simulink model "BugE_v0_40_MAS_loads_reg"  (R2015b)
settings: Solver=FixedStepDiscrete  StartTime=0.0  StopTime=1370  FixedStep=sample_time  RelTol=1e-3
values from neighbouring files (symbols this model uses):
  AB_diode_dV = 0.9    [main_sync.m]
  air_density = 1.225    [main_sync.m]
  bus_ac_Pmax_abs = 240    [main_sync.m]
  bus_charger_Pmax = 1000    [main_sync.m]
  bus_load_Pmax_abs = 260    [main_sync.m]
  capInitVolt = capVmax*sqrt(capInitSoC)    [main_sync.m]
  cyc_kph = [cyc_kph(:,1), cyc_kph(:,2)*speed_max_limit/speed_max]    [main_sync.m]
  cyc_repeat = 0    [main_sync.m]
  ess1_init_soc = 1    [main_sync.m]
  ess1_soh = 1    [main_sync.m]
  ess2_init_soc = 1    [main_sync.m]
  ess2_soh = 1    [main_sync.m]
  ess3_init_soc = 1    [main_sync.m]
  ess3_soh = 1    [main_sync.m]
  ess4_init_soc = 1    [main_sync.m]
  ess4_soh = 1    [main_sync.m]
  ess5_init_soc = 1    [main_sync.m]
  ess5_soh = 1    [main_sync.m]
  gear_ratio = 6    [main_sync.m]
  JADE_on = 0    [main_sync.m]
  loadpower = rawcsv(:,2)    [main_sync.m]
  loadtime = rawcsv(:,1)    [main_sync.m]
  lockSOCs = 0    [main_sync.m]
  max_brk_torque = 300    [main_sync.m]
  no_wheels = 3    [main_sync.m]
  period2 = max(loadtime)    [main_sync.m]
  PV_Pmax = 100    [main_sync.m]
  sample_time = 0.01    [main_sync.m]
  startup_seq_step_delay = 0.2    [main_sync.m]
  stop_option = 0    [main_sync.m]
  use_drive_cycle = 1    [main_sync.m]
  use_real_subs_loads = 1    [main_sync.m]
  vbus_max = 25    [main_sync.m]
  vbus_min = 17    [main_sync.m]
  vbus_safety_threshold = 2    [main_sync.m]
  vbus_threshold = 20    [main_sync.m]
  veh_CD = 0.35    [main_sync.m]
  veh_FA = 1.543    [main_sync.m]
  veh_gravity = 9.81*veh_mass    (= 1863.9)    [main_sync.m]
  veh_mass = 190    [main_sync.m]
  wh_1st_rrc = 0.02    [main_sync.m]
  wh_bearing_frc = 0.0015    [main_sync.m]
  wh_inertia = 0.0556    [main_sync.m]
  wh_radius = 0.508/2    (= 0.254)    [main_sync.m]
undefined symbols (not defined in the file or in its folder): capC, capR, cyc_acc, cyc_avg_time_samples, cyc_brk, cyc_grade, cyc_key, DCM_eff_factor_for_Vin, DCM_eff_for_Iout, DCM_Iout, DCM_Iout_max, DCM_Pin_noload, DCM_Pout_max, DCM_Vin, DCM_Vout, DiscIntNeverNeededParam, ess2_coulombic_eff, ess2_Ineg_max_SOC, ess2_Ineg_max_temp, ess2_Ipos_max_SOC, ess2_Ipos_max_temp, ess2_max_ah_cap, ess2_max_volts, ess2_min_volts, ess2_module_parallel, ess2_module_series, ess2_r_dis, ess2_soc, ess2_SOC_for_Ilimit, ess2_temp_for_Ilimit, ess2_temp_max, ess2_tmp, ess2_voc, ess3_coulombic_eff, ess3_max_ah_cap, ess3_module_parallel, ess3_module_series, ess3_r_dis, ess3_soc, ess3_tmp, ess3_voc, ess_coulombic_eff, ess_Ineg_max_SOC, ess_Ineg_max_temp, ess_Ipos_max_SOC, ess_Ipos_max_temp, ess_max_ah_cap, ess_max_volts, ess_min_volts, ess_module_parallel, ess_module_series, ess_nominal_volts, ess_r_dis, ess_soc, ess_SOC_for_Ilimit, ess_temp_for_Ilimit, ess_temp_max, ess_tmp, ess_voc, MC_eff1 ... (+18)
libraries: simulink x140, commfilt2 x1, simulink_extras x1
(part 4 of 7)

== system BugE_v0_40_MAS_loads_reg/Energy Storage (New Grid)/MB2 DCDC/eff_maps ==
  "P into bus cmd " : Inport
  Vbus : Inport  Port=2
  Vbatt : Inport  Port=3
  1/V : Product  Inputs=*/
  >= eps : Saturate  UpperLimit=inf  LowerLimit=eps
  Clock : Clock
  Demux : Demux  Outputs=2
  Discrete-Time Integrator : DiscreteIntegrator  InitialConditionSetting=State (most efficient)  SampleTime=sample_time  ICPrevOutput=DiscIntNeverNeededParam  ICPrevScaledInput=DiscIntNeverNeededParam
  Discrete-Time Integrator1 : DiscreteIntegrator  InitialConditionSetting=State (most efficient)  SampleTime=sample_time  ICPrevOutput=DiscIntNeverNeededParam  ICPrevScaledInput=DiscIntNeverNeededParam
  Display : Display
  Divide : Product  Inputs=/*
  Divide1 : Product  Inputs=*/
  Gain : Gain  Gain=-1
  Interpolation: efficiency2 : Lookup_n-D  NumberOfTableDimensions=3  BreakpointsForDimension1=MC_Pouts  BreakpointsForDimension2=MC_Vins  BreakpointsForDimension3=MC_Vouts  Table=MC_eff2  InterpMethod=Cubic spline  InternalRulePriority=Speed  RndMeth=Simplest  InputSameDT=on
  Interpolation: efficiency1 : Lookup_n-D  NumberOfTableDimensions=3  BreakpointsForDimension1=MC_Pins  BreakpointsForDimension2=MC_Vins  BreakpointsForDimension3=MC_Vouts  Table=MC_eff1  InterpMethod=Cubic spline  InternalRulePriority=Speed  RndMeth=Simplest  InputSameDT=on
  Mux : Mux  Inputs=2
  Mux1 : Mux  Inputs=2
  Mux2 : Mux  Inputs=2
  P from batt : Switch
  P from batt1 : Switch
  Product : Product
  Saturation : Saturate  UpperLimit=MC_max_eff  LowerLimit=eps
  Saturation1 : Saturate  UpperLimit=MC_max_eff  LowerLimit=eps
  Saturation2 : Saturate  UpperLimit=inf  LowerLimit=eps
  Subtract : Sum  Inputs=+-
  Switch1 : Switch
  avg eff : Display
  I from batt & into bus : Outport
  wires:
  Vbatt/1 -> Mux/2, Mux1/1
  Demux/2 -> Interpolation: efficiency1/3, Interpolation: efficiency2/3
  Mux/1 -> Switch1/3
  Switch1/1 -> Demux/1
  Gain/1 -> Interpolation: efficiency1/1
  Divide/1 -> P from batt/1
  Interpolation: efficiency1/1 -> Saturation1/1
  Product/1 -> P from batt/3
  Mux2/1 -> 1/V/1
  Mux1/1 -> >= eps/1, Switch1/1
  1/V/1 -> I from batt & into bus/1
  >= eps/1 -> 1/V/2
  Demux/1 -> Interpolation: efficiency2/2, Interpolation: efficiency1/2
  Vbus/1 -> Mux1/2, Mux/1
  Saturation/1 -> Divide/1
  P from batt/1 -> Subtract/1, Mux2/1
  Subtract/1 -> Discrete-Time Integrator/1
  Discrete-Time Integrator/1 -> Display/1  "E lost MB2 DCDC"
  Interpolation: efficiency2/1 -> P from batt1/1, Saturation/1
  "P into bus cmd "/1 -> Subtract/2, Gain/1, Interpolation: efficiency2/1, Switch1/2, Divide/2, Product/1, P from batt1/2, P from batt/2, Mux2/2
  Saturation1/1 -> P from batt1/3, Product/2
  P from batt1/1 -> Discrete-Time Integrator1/1
  Discrete-Time Integrator1/1 -> Divide1/1
  Clock/1 -> Saturation2/1
  Divide1/1 -> avg eff/1
  Saturation2/1 -> Divide1/2

== system BugE_v0_40_MAS_loads_reg/Energy Storage (New Grid)/MB2 DCDC/eff_maps1 ==
  I motor : Inport
  Vbatt cmd : Inport  Port=2
  Vbus : Inport  Port=3
  >= eps : Saturate  UpperLimit=inf  LowerLimit=eps
  Gain : Gain  Gain=-1
  I from bus : Product  Inputs=*//
  Interpolation: efficiency2 : Lookup_n-D  NumberOfTableDimensions=3  BreakpointsForDimension1=MC_Pouts  BreakpointsForDimension2=MC_Vins  BreakpointsForDimension3=MC_Vouts  Table=MC_eff2  InterpMethod=Cubic spline  InternalRulePriority=Speed  RndMeth=Simplest  InputSameDT=on
  Mux2 : Mux  Inputs=2
  P out to motor : Product
  Saturation : Saturate  UpperLimit=MC_max_eff  LowerLimit=eps
  I from batt & into bus : Outport
  wires:
  Interpolation: efficiency2/1 -> Saturation/1
  Mux2/1 -> Gain/1
  Gain/1 -> I from batt & into bus/1
  Vbus/1 -> >= eps/1
  Vbatt cmd/1 -> Interpolation: efficiency2/3, P out to motor/2
  I motor/1 -> Mux2/1, P out to motor/1
  P out to motor/1 -> Interpolation: efficiency2/1, I from bus/1
  I from bus/1 -> Mux2/2
  >= eps/1 -> I from bus/3, Interpolation: efficiency2/2
  Saturation/1 -> I from bus/2

== system BugE_v0_40_MAS_loads_reg/Energy Storage (New Grid)/PV_cells Pout/Energy Quantification ==
  Power : Inport
  tag scope: E_PV=global
  wires:
  Power/1 -> [E_PV]

== system BugE_v0_40_MAS_loads_reg/Energy Storage (New Grid)/SB1/Calculate SOC ==
  Temp [C] : Inport
  I [A] : Inport  Port=2
  1/3600 : Gain  Gain=1/3600
  Add : Sum  Inputs=-+
  Constant1 : Constant  SampleTime=sample_time
  Coulombic efficiency : Lookup_n-D  NumberOfTableDimensions=1  BreakpointsForDimension1=ess2_tmp  Table=ess2_coulombic_eff  InternalRulePriority=Speed  SaturateOnIntegerOverflow=on  InputSameDT=on
  Energy used [Ah] : DiscreteIntegrator  InitialConditionSource=external  InitialConditionSetting=State (most efficient)  SampleTime=sample_time  ICPrevOutput=DiscIntNeverNeededParam  ICPrevScaledInput=DiscIntNeverNeededParam
  Energy left [Ah] : Sum  Inputs=-+
  I adjusted : Product
  Max capacity [Ah] w/ SOH : Lookup_n-D  NumberOfTableDimensions=1  BreakpointsForDimension1=ess2_tmp  Table=ess2_max_ah_cap*ess3_soh  InternalRulePriority=Speed  SaturateOnIntegerOverflow=on  InputSameDT=on
  Multiply : Product
  Multiply1 : Product
  "SOC " : Product  Inputs=*/
  Saturation : Saturate  UpperLimit=1  LowerLimit=0
  Switch : Switch  Criteria=u2 > Threshold
  Switch1 : Switch  Criteria=u2 > Threshold
  ess2_modules : Constant  Value=ess2_module_series*ess2_module_parallel  SampleTime=sample_time
  ess3_init_soc : Constant  Value=ess3_init_soc  SampleTime=sample_time
  lockSOCs : Constant  Value=lockSOCs
  SOC : Outport
  wires:
  Energy used [Ah]/1 -> Energy left [Ah]/1
  I [A]/1 -> Switch/2, Switch/1, I adjusted/1
  Switch/1 -> 1/3600/1
  Coulombic efficiency/1 -> I adjusted/2
  Energy left [Ah]/1 -> "SOC "/1
  I adjusted/1 -> Switch/3
  1/3600/1 -> Energy used [Ah]/1
  Temp [C]/1 -> Max capacity [Ah] w/ SOH/1, Coulombic efficiency/1
  Multiply1/1 -> Multiply/2, "SOC "/2, Energy left [Ah]/2
  "SOC "/1 -> Saturation/1
  Constant1/1 -> Add/2
  Multiply/1 -> Energy used [Ah]/2
  Add/1 -> Multiply/1
  ess2_modules/1 -> Multiply1/2
  Max capacity [Ah] w/ SOH/1 -> Multiply1/1
  ess3_init_soc/1 -> Switch1/1, Add/1
  Saturation/1 -> Switch1/3
  lockSOCs/1 -> Switch1/2
  Switch1/1 -> SOC/1

== system BugE_v0_40_MAS_loads_reg/Energy Storage (New Grid)/SB1/Compute current (nolimit) ==
  Voc [V] : Inport
  Rint [Ohm] : Inport  Port=2
  Output power [W] : Inport  Port=3
  2*R : Gain  Gain=2
  4*R*Pbty : Gain  Gain=4
  I*R : Product  Inputs=**
  Ibty : Product  Inputs=*/
  R*Pbty : Product
  Sqrt : Sqrt  SaturateOnIntegerOverflow=on
  "Voc-I*R " : Sum  Inputs=+-
  Voc-sqrt : Sum  Inputs=+-
  Voc^2 : Product
  Voc^2 -4R*Pbty : Sum  Inputs=+-
  I [A] : Outport
  V [V] : Outport  Port=2
  wires:
  Output power [W]/1 -> R*Pbty/1
  Voc [V]/1 -> "Voc-I*R "/1, Voc-sqrt/1, Voc^2/2, Voc^2/1
  Rint [Ohm]/1 -> R*Pbty/2, 2*R/1, I*R/2
  R*Pbty/1 -> 4*R*Pbty/1
  Voc^2/1 -> Voc^2 -4R*Pbty/1
  4*R*Pbty/1 -> Voc^2 -4R*Pbty/2
  Voc^2 -4R*Pbty/1 -> Sqrt/1
  Sqrt/1 -> Voc-sqrt/2
  Voc-sqrt/1 -> Ibty/1
  2*R/1 -> Ibty/2
  Ibty/1 -> I [A]/1, I*R/1
  I*R/1 -> "Voc-I*R "/2
  "Voc-I*R "/1 -> V [V]/1

== system BugE_v0_40_MAS_loads_reg/Energy Storage (New Grid)/SB1/Energy Quantification ==
  In2 : Inport
  In3 : Inport  Port=2
  In1 : Inport  Port=3
  < 0 : Saturate  UpperLimit=0  LowerLimit=-inf
  > 0 : Saturate  UpperLimit=inf  LowerLimit=0  LinearizeAsGain=off
  Gain : Gain  Gain=-1
  Power : Product
  power loss : Product  Inputs=3
  tag scope: E_batt_loss3=global, E_batt_regen3=global, E_batt_useful3=global
  wires:
  In2/1 -> Power/1
  In3/1 -> Power/2, power loss/2, power loss/1
  Gain/1 -> [E_batt_regen3]
  Power/1 -> < 0/1, > 0/1
  < 0/1 -> Gain/1
  > 0/1 -> [E_batt_useful3]
  power loss/1 -> [E_batt_loss3]
  In1/1 -> power loss/3

== system BugE_v0_40_MAS_loads_reg/Energy Storage (New Grid)/SB1/Pack Voc, R ==
  SOC_prev : Inport
  Req. power [W] : Inport  Port=2
  Temp [degC] : Inport  Port=3
  >=0 : simulink/Logic and Bit Operations/Compare To Zero  relop=>=  OutDataTypeStr=boolean
  Product : Product  Inputs=3
  Product1 : Product  Inputs=/**/
  Product2 : Product  Inputs=/**/
  R_charge [Ohm] : Lookup_n-D  BreakpointsForDimension1=ess2_tmp  BreakpointsForDimension2=ess2_soc  Table=ess2_r_dis  InternalRulePriority=Speed  RndMeth=Simplest  InputSameDT=on
  R_discharge [Ohm] : Lookup_n-D  BreakpointsForDimension1=ess2_tmp  BreakpointsForDimension2=ess2_soc  Table=ess2_r_dis  InternalRulePriority=Speed  RndMeth=Simplest  InputSameDT=on
  Switch : Switch  Criteria=u2 > Threshold
  VOC [V] : Lookup_n-D  BreakpointsForDimension1=ess2_tmp  BreakpointsForDimension2=ess2_soc  Table=ess2_voc  InternalRulePriority=Speed  RndMeth=Simplest  InputSameDT=on
  ess2_module _parallel : Constant  Value=ess2_module_parallel  SampleTime=sample_time
  ess2_module _series : Constant  Value=ess2_module_series  SampleTime=sample_time
  ess3_soh : Constant  Value=ess3_soh  SampleTime=sample_time
  Pack Voc [V] : Outport
  Pack R [Ohm] : Outport  Port=2
  wires:
  Switch/1 -> Pack R [Ohm]/1
  Req. power [W]/1 -> >=0/1
  R_discharge [Ohm]/1 -> Product1/2
  Product/1 -> Pack Voc [V]/1
  VOC [V]/1 -> Product/2
  ess2_module _series/1 -> Product/3, Product2/2, Product1/3
  Temp [degC]/1 -> R_charge [Ohm]/1, R_discharge [Ohm]/1, VOC [V]/1
  SOC_prev/1 -> R_charge [Ohm]/2, R_discharge [Ohm]/2, VOC [V]/2
  ess3_soh/1 -> Product2/1, Product1/1, Product/1
  >=0/1 -> Switch/2
  ess2_module _parallel/1 -> Product1/4, Product2/4
  R_charge [Ohm]/1 -> Product2/3
  Product2/1 -> Switch/3
  Product1/1 -> Switch/1

== system BugE_v0_40_MAS_loads_reg/Energy Storage (New Grid)/SB1 DCDC/Current limiter ==
  enable DCDC : Inport
  I batt side raw : Inport  Port=2
  I bus side raw : Inport  Port=3
  I max : Inport  Port=4
  " ==0 " : simulink/Logic and Bit Operations/Compare To Zero  relop===  OutDataTypeStr=boolean
  0 : Constant  Value=0  SampleTime=sample_time
  ==0 : simulink/Logic and Bit Operations/Compare To Zero  relop===  OutDataTypeStr=boolean
  Abs : Abs
  Abs1 : Abs
  Constant : Constant  SampleTime=sample_time
  Iin final : Product  Inputs=**
  Iin limited : Switch  Criteria=u2 > Threshold
  Iin over limit : RelationalOperator  Operator=>  OutDataTypeStr=boolean
  Iin raw avoid 0 div : Switch  Criteria=u2 > Threshold
  Imax : Product
  Iout final : Product  Inputs=**
  Iout limited : Switch  Criteria=u2 > Threshold
  Iout over limit : RelationalOperator  Operator=<  OutDataTypeStr=boolean
  Iout raw avoid 0 div : Switch  Criteria=u2 > Threshold
  Sign : Signum
  avoid 0 div2 : Switch  Criteria=u2 > Threshold
  avoid 0 div3 : Switch  Criteria=u2 > Threshold
  disable : Logic  Operator=NOT  AllPortsSameDT=off  OutDataTypeStr=boolean
  limit ratio : MinMax  Inputs=2
  limit ratio1 : Product  Inputs=*/
  limit ratio2 : Product  Inputs=*/
  or : Logic  Operator=OR  Inputs=3  AllPortsSameDT=off  OutDataTypeStr=boolean
  I batt side lim : Outport
  I bus side lim : Outport  Port=2
  wires:
  Iout raw avoid 0 div/1 -> Abs1/1, Iout final/2, limit ratio2/2, Iout limited/3
  Iin raw avoid 0 div/1 -> limit ratio1/2, Iin final/1, Iin limited/3, Sign/1, Abs/1
  Iin final/1 -> avoid 0 div2/3
  limit ratio2/1 -> limit ratio/2
  avoid 0 div3/1 -> I bus side lim/1
  Iin over limit/1 -> Iin limited/2
  Iout limited/1 -> limit ratio2/1
  Abs1/1 -> Iout over limit/2
  I max/1 -> Iin over limit/2, Imax/2, Iout over limit/1
  limit ratio/1 -> Iin final/2, Iout final/1
  Imax/1 -> Iin limited/1, Iout limited/1
  Abs/1 -> Iin over limit/1
  Sign/1 -> Imax/1
  limit ratio1/1 -> limit ratio/1
  Iin limited/1 -> limit ratio1/1
  Iout over limit/1 -> Iout limited/2
  I batt side raw/1 -> " ==0 "/1, Iin raw avoid 0 div/3
  enable DCDC/1 -> disable/1
  Constant/1 -> Iout raw avoid 0 div/1, Iin raw avoid 0 div/1
  I bus side raw/1 -> ==0/1, Iout raw avoid 0 div/3
  Iout final/1 -> avoid 0 div3/3
  0/1 -> avoid 0 div2/1, avoid 0 div3/1
  avoid 0 div2/1 -> I batt side lim/1
  or/1 -> avoid 0 div3/2, avoid 0 div2/2, Iin raw avoid 0 div/2, Iout raw avoid 0 div/2
  disable/1 -> or/3
  ==0/1 -> or/2
  " ==0 "/1 -> or/1

== system BugE_v0_40_MAS_loads_reg/Energy Storage (New Grid)/SB1 DCDC/Energy Quantification ==
  In1 : Inport
  In2 : Inport  Port=2
  In3 : Inport  Port=3
  In4 : Inport  Port=4
  Abs : Abs
  P lost : Sum  Inputs=-+
  Pin_DAB : Product
  Pout_DAB : Product
  tag scope: E_DAB3_loss=global
  wires:
  P lost/1 -> Abs/1
  In3/1 -> Pin_DAB/1
  Abs/1 -> [E_DAB3_loss]
  Pin_DAB/1 -> P lost/2
  Pout_DAB/1 -> P lost/1
  In4/1 -> Pin_DAB/2
  In2/1 -> Pout_DAB/2
  In1/1 -> Pout_DAB/1

== system BugE_v0_40_MAS_loads_reg/Energy Storage (New Grid)/SB1 DCDC/eff_maps1 ==
  "P into bus cmd " : Inport
  Vbus : Inport  Port=2
  Vbatt : Inport  Port=3
  1/V : Product  Inputs=*/
  >= eps : Saturate  UpperLimit=inf  LowerLimit=eps
  Demux : Demux  Outputs=2
  Divide : Product  Inputs=/*
  Gain : Gain  Gain=-1
  Interpolation: efficiency2 : Lookup_n-D  NumberOfTableDimensions=3  BreakpointsForDimension1=MC_Pouts  BreakpointsForDimension2=MC_Vins  BreakpointsForDimension3=MC_Vouts  Table=MC_eff2  InterpMethod=Cubic spline  InternalRulePriority=Speed  RndMeth=Simplest  InputSameDT=on
  Interpolation: efficiency1 : Lookup_n-D  NumberOfTableDimensions=3  BreakpointsForDimension1=MC_Pins  BreakpointsForDimension2=MC_Vins  BreakpointsForDimension3=MC_Vouts  Table=MC_eff1  InterpMethod=Cubic spline  InternalRulePriority=Speed  RndMeth=Simplest  InputSameDT=on
  Mux : Mux  Inputs=2
  Mux1 : Mux  Inputs=2
  Mux2 : Mux  Inputs=2
  P from batt : Switch
  Product : Product
  Saturation : Saturate  UpperLimit=MC_max_eff  LowerLimit=eps
  Saturation1 : Saturate  UpperLimit=MC_max_eff  LowerLimit=eps
  Switch1 : Switch
  I from batt & into bus : Outport
  wires:
  Vbus/1 -> Mux1/2, Mux/1
  Vbatt/1 -> Mux/2, Mux1/1
  Demux/2 -> Interpolation: efficiency1/3, Interpolation: efficiency2/3
  Mux/1 -> Switch1/3
  Switch1/1 -> Demux/1
  Gain/1 -> Interpolation: efficiency1/1
  Interpolation: efficiency2/1 -> Saturation/1
  Divide/1 -> P from batt/1
  Interpolation: efficiency1/1 -> Saturation1/1
  Product/1 -> P from batt/3
  P from batt/1 -> Mux2/1
  "P into bus cmd "/1 -> Gain/1, Interpolation: efficiency2/1, Switch1/2, Divide/2, Product/1, P from batt/2, Mux2/2
  Mux2/1 -> 1/V/1
  Mux1/1 -> >= eps/1, Switch1/1
  1/V/1 -> I from batt & into bus/1
  >= eps/1 -> 1/V/2
  Saturation/1 -> Divide/1
  Saturation1/1 -> Product/2
  Demux/1 -> Interpolation: efficiency2/2, Interpolation: efficiency1/2

== system BugE_v0_40_MAS_loads_reg/Energy Storage (New Grid)/SB2/Calculate SOC ==
  Temp [C] : Inport
  I [A] : Inport  Port=2
  1/3600 : Gain  Gain=1/3600
  Add : Sum  Inputs=-+
  Constant1 : Constant  SampleTime=sample_time
  Coulombic efficiency : Lookup_n-D  NumberOfTableDimensions=1  BreakpointsForDimension1=ess2_tmp  Table=ess2_coulombic_eff  InternalRulePriority=Speed  SaturateOnIntegerOverflow=on  InputSameDT=on
  Energy used [Ah] : DiscreteIntegrator  InitialConditionSource=external  InitialConditionSetting=State (most efficient)  SampleTime=sample_time  ICPrevOutput=DiscIntNeverNeededParam  ICPrevScaledInput=DiscIntNeverNeededParam
  Energy left [Ah] : Sum  Inputs=-+
  I adjusted : Product
  Max capacity [Ah] w/ SOH : Lookup_n-D  NumberOfTableDimensions=1  BreakpointsForDimension1=ess2_tmp  Table=ess2_max_ah_cap*ess4_soh  InternalRulePriority=Speed  SaturateOnIntegerOverflow=on  InputSameDT=on
  Multiply : Product
  Multiply1 : Product
  "SOC " : Product  Inputs=*/
  Saturation : Saturate  UpperLimit=1  LowerLimit=0
  Switch : Switch  Criteria=u2 > Threshold
  Switch1 : Switch  Criteria=u2 > Threshold
  ess2_modules : Constant  Value=ess2_module_series*ess2_module_parallel  SampleTime=sample_time
  ess3_init_soc : Constant  Value=ess4_init_soc  SampleTime=sample_time
  lockSOCs : Constant  Value=lockSOCs
  SOC : Outport
  wires:
  Energy used [Ah]/1 -> Energy left [Ah]/1
  I [A]/1 -> Switch/2, Switch/1, I adjusted/1
  Switch/1 -> 1/3600/1
  Coulombic efficiency/1 -> I adjusted/2
  Energy left [Ah]/1 -> "SOC "/1
  I adjusted/1 -> Switch/3
  1/3600/1 -> Energy used [Ah]/1
  Temp [C]/1 -> Max capacity [Ah] w/ SOH/1, Coulombic efficiency/1
  Multiply1/1 -> Multiply/2, "SOC "/2, Energy left [Ah]/2
  "SOC "/1 -> Saturation/1
  Constant1/1 -> Add/2
  Multiply/1 -> Energy used [Ah]/2
  Add/1 -> Multiply/1
  ess2_modules/1 -> Multiply1/2
  Max capacity [Ah] w/ SOH/1 -> Multiply1/1
  ess3_init_soc/1 -> Switch1/1, Add/1
  Saturation/1 -> Switch1/3
  lockSOCs/1 -> Switch1/2
  Switch1/1 -> SOC/1

== system BugE_v0_40_MAS_loads_reg/Energy Storage (New Grid)/SB2/Compute current (nolimit) ==
  Voc [V] : Inport
  Rint [Ohm] : Inport  Port=2
  Output power [W] : Inport  Port=3
  2*R : Gain  Gain=2
  4*R*Pbty : Gain  Gain=4
  I*R : Product  Inputs=**
  Ibty : Product  Inputs=*/
  R*Pbty : Product
  Sqrt : Sqrt  SaturateOnIntegerOverflow=on
  "Voc-I*R " : Sum  Inputs=+-
  Voc-sqrt : Sum  Inputs=+-
  Voc^2 : Product
  Voc^2 -4R*Pbty : Sum  Inputs=+-
  I [A] : Outport
  V [V] : Outport  Port=2
  wires:
  Output power [W]/1 -> R*Pbty/1
  Voc [V]/1 -> "Voc-I*R "/1, Voc-sqrt/1, Voc^2/2, Voc^2/1
  Rint [Ohm]/1 -> R*Pbty/2, 2*R/1, I*R/2
  R*Pbty/1 -> 4*R*Pbty/1
  Voc^2/1 -> Voc^2 -4R*Pbty/1
  4*R*Pbty/1 -> Voc^2 -4R*Pbty/2
  Voc^2 -4R*Pbty/1 -> Sqrt/1
  Sqrt/1 -> Voc-sqrt/2
  Voc-sqrt/1 -> Ibty/1
  2*R/1 -> Ibty/2
  Ibty/1 -> I [A]/1, I*R/1
  I*R/1 -> "Voc-I*R "/2
  "Voc-I*R "/1 -> V [V]/1

== system BugE_v0_40_MAS_loads_reg/Energy Storage (New Grid)/SB2/Energy Quantification ==
  In2 : Inport
  In3 : Inport  Port=2
  In1 : Inport  Port=3
  < 0 : Saturate  UpperLimit=0  LowerLimit=-inf
  > 0 : Saturate  UpperLimit=inf  LowerLimit=0  LinearizeAsGain=off
  Gain : Gain  Gain=-1
  Power : Product
  power loss : Product  Inputs=3
  tag scope: E_batt_loss4=global, E_batt_regen4=global, E_batt_useful4=global
  wires:
  In2/1 -> Power/1
  In3/1 -> Power/2, power loss/2, power loss/1
  Gain/1 -> [E_batt_regen4]
  Power/1 -> < 0/1, > 0/1
  < 0/1 -> Gain/1
  > 0/1 -> [E_batt_useful4]
  power loss/1 -> [E_batt_loss4]
  In1/1 -> power loss/3

== system BugE_v0_40_MAS_loads_reg/Energy Storage (New Grid)/SB2/Pack Voc, R ==
  SOC_prev : Inport
  Req. power [W] : Inport  Port=2
  Temp [degC] : Inport  Port=3
  >=0 : simulink/Logic and Bit Operations/Compare To Zero  relop=>=  OutDataTypeStr=boolean
  Product : Product  Inputs=3
  Product1 : Product  Inputs=/**/
  Product2 : Product  Inputs=/**/
  R_charge [Ohm] : Lookup_n-D  BreakpointsForDimension1=ess2_tmp  BreakpointsForDimension2=ess2_soc  Table=ess2_r_dis  InternalRulePriority=Speed  RndMeth=Simplest  InputSameDT=on
  R_discharge [Ohm] : Lookup_n-D  BreakpointsForDimension1=ess2_tmp  BreakpointsForDimension2=ess2_soc  Table=ess2_r_dis  InternalRulePriority=Speed  RndMeth=Simplest  InputSameDT=on
  Switch : Switch  Criteria=u2 > Threshold
  VOC [V] : Lookup_n-D  BreakpointsForDimension1=ess2_tmp  BreakpointsForDimension2=ess2_soc  Table=ess2_voc  InternalRulePriority=Speed  RndMeth=Simplest  InputSameDT=on
  ess2_module _parallel : Constant  Value=ess2_module_parallel  SampleTime=sample_time
  ess2_module _series : Constant  Value=ess2_module_series  SampleTime=sample_time
  ess3_soh : Constant  Value=ess3_soh  SampleTime=sample_time
  Pack Voc [V] : Outport
  Pack R [Ohm] : Outport  Port=2
  wires:
  Switch/1 -> Pack R [Ohm]/1
  Req. power [W]/1 -> >=0/1
  R_discharge [Ohm]/1 -> Product1/2
  Product/1 -> Pack Voc [V]/1
  VOC [V]/1 -> Product/2
  ess2_module _series/1 -> Product/3, Product2/2, Product1/3
  Temp [degC]/1 -> R_charge [Ohm]/1, R_discharge [Ohm]/1, VOC [V]/1
  SOC_prev/1 -> R_charge [Ohm]/2, R_discharge [Ohm]/2, VOC [V]/2
  ess3_soh/1 -> Product2/1, Product1/1, Product/1
  >=0/1 -> Switch/2
  ess2_module _parallel/1 -> Product1/4, Product2/4
  R_charge [Ohm]/1 -> Product2/3
  Product2/1 -> Switch/3
  Product1/1 -> Switch/1

== system BugE_v0_40_MAS_loads_reg/Energy Storage (New Grid)/SB2 DCDC/Current limiter ==
  enable DCDC : Inport
  I batt side raw : Inport  Port=2
  I bus side raw : Inport  Port=3
  I max : Inport  Port=4
  " ==0 " : simulink/Logic and Bit Operations/Compare To Zero  relop===  OutDataTypeStr=boolean
  0 : Constant  Value=0  SampleTime=sample_time
  ==0 : simulink/Logic and Bit Operations/Compare To Zero  relop===  OutDataTypeStr=boolean
  Abs : Abs
  Abs1 : Abs
  Constant : Constant  SampleTime=sample_time
  Iin final : Product  Inputs=**
  Iin limited : Switch  Criteria=u2 > Threshold
  Iin over limit : RelationalOperator  Operator=>  OutDataTypeStr=boolean
  Iin raw avoid 0 div : Switch  Criteria=u2 > Threshold
  Imax : Product
  Iout final : Product  Inputs=**
  Iout limited : Switch  Criteria=u2 > Threshold
  Iout over limit : RelationalOperator  Operator=<  OutDataTypeStr=boolean
  Iout raw avoid 0 div : Switch  Criteria=u2 > Threshold
  Sign : Signum
  avoid 0 div2 : Switch  Criteria=u2 > Threshold
  avoid 0 div3 : Switch  Criteria=u2 > Threshold
  disable : Logic  Operator=NOT  AllPortsSameDT=off  OutDataTypeStr=boolean
  limit ratio : MinMax  Inputs=2
  limit ratio1 : Product  Inputs=*/
  limit ratio2 : Product  Inputs=*/
  or : Logic  Operator=OR  Inputs=3  AllPortsSameDT=off  OutDataTypeStr=boolean
  I batt side lim : Outport
  I bus side lim : Outport  Port=2
  wires:
  Iout raw avoid 0 div/1 -> Abs1/1, Iout final/2, limit ratio2/2, Iout limited/3
  Iin raw avoid 0 div/1 -> limit ratio1/2, Iin final/1, Iin limited/3, Sign/1, Abs/1
  Iin final/1 -> avoid 0 div2/3
  limit ratio2/1 -> limit ratio/2
  avoid 0 div3/1 -> I bus side lim/1
  Iin over limit/1 -> Iin limited/2
  Iout limited/1 -> limit ratio2/1
  Abs1/1 -> Iout over limit/2
  I max/1 -> Iin over limit/2, Imax/2, Iout over limit/1
  limit ratio/1 -> Iin final/2, Iout final/1
  Imax/1 -> Iin limited/1, Iout limited/1
  Abs/1 -> Iin over limit/1
  Sign/1 -> Imax/1
  limit ratio1/1 -> limit ratio/1
  Iin limited/1 -> limit ratio1/1
  Iout over limit/1 -> Iout limited/2
  I batt side raw/1 -> " ==0 "/1, Iin raw avoid 0 div/3
  enable DCDC/1 -> disable/1
  Constant/1 -> Iout raw avoid 0 div/1, Iin raw avoid 0 div/1
  I bus side raw/1 -> ==0/1, Iout raw avoid 0 div/3
  Iout final/1 -> avoid 0 div3/3
  0/1 -> avoid 0 div2/1, avoid 0 div3/1
  avoid 0 div2/1 -> I batt side lim/1
  or/1 -> avoid 0 div3/2, avoid 0 div2/2, Iin raw avoid 0 div/2, Iout raw avoid 0 div/2
  disable/1 -> or/3
  ==0/1 -> or/2
  " ==0 "/1 -> or/1

== system BugE_v0_40_MAS_loads_reg/Energy Storage (New Grid)/SB2 DCDC/Energy Quantification ==
  In1 : Inport
  In2 : Inport  Port=2
  In3 : Inport  Port=3
  In4 : Inport  Port=4
  Abs : Abs
  P lost : Sum  Inputs=-+
  Pin_DAB : Product
  Pout_DAB : Product
  tag scope: E_DAB4_loss=global
  wires:
  P lost/1 -> Abs/1
  In3/1 -> Pin_DAB/1
  Abs/1 -> [E_DAB4_loss]
  Pin_DAB/1 -> P lost/2
  Pout_DAB/1 -> P lost/1
  In4/1 -> Pin_DAB/2
  In2/1 -> Pout_DAB/2
  In1/1 -> Pout_DAB/1

== system BugE_v0_40_MAS_loads_reg/Energy Storage (New Grid)/SB2 DCDC/eff_maps1 ==
  "P into bus cmd " : Inport
  Vbus : Inport  Port=2
  Vbatt : Inport  Port=3
  1/V : Product  Inputs=*/
  >= eps : Saturate  UpperLimit=inf  LowerLimit=eps
  Demux : Demux  Outputs=2
  Divide : Product  Inputs=/*
  Gain : Gain  Gain=-1
  Interpolation: efficiency2 : Lookup_n-D  NumberOfTableDimensions=3  BreakpointsForDimension1=MC_Pouts  BreakpointsForDimension2=MC_Vins  BreakpointsForDimension3=MC_Vouts  Table=MC_eff2  InterpMethod=Cubic spline  InternalRulePriority=Speed  RndMeth=Simplest  InputSameDT=on
  Interpolation: efficiency1 : Lookup_n-D  NumberOfTableDimensions=3  BreakpointsForDimension1=MC_Pins  BreakpointsForDimension2=MC_Vins  BreakpointsForDimension3=MC_Vouts  Table=MC_eff1  InterpMethod=Cubic spline  InternalRulePriority=Speed  RndMeth=Simplest  InputSameDT=on
  Mux : Mux  Inputs=2
  Mux1 : Mux  Inputs=2
  Mux2 : Mux  Inputs=2
  P from batt : Switch
  Product : Product
  Saturation : Saturate  UpperLimit=MC_max_eff  LowerLimit=eps
  Saturation1 : Saturate  UpperLimit=MC_max_eff  LowerLimit=eps
  Switch1 : Switch
  I from batt & into bus : Outport
  wires:
  Vbus/1 -> Mux1/2, Mux/1
  Vbatt/1 -> Mux/2, Mux1/1
  Demux/2 -> Interpolation: efficiency1/3, Interpolation: efficiency2/3
  Mux/1 -> Switch1/3
  Switch1/1 -> Demux/1
  Gain/1 -> Interpolation: efficiency1/1
  Interpolation: efficiency2/1 -> Saturation/1
  Divide/1 -> P from batt/1
  Interpolation: efficiency1/1 -> Saturation1/1
  Product/1 -> P from batt/3
  P from batt/1 -> Mux2/1
  "P into bus cmd "/1 -> Gain/1, Interpolation: efficiency2/1, Switch1/2, Divide/2, Product/1, P from batt/2, Mux2/2
  Mux2/1 -> 1/V/1
  Mux1/1 -> >= eps/1, Switch1/1
  1/V/1 -> I from batt & into bus/1
  >= eps/1 -> 1/V/2
  Saturation/1 -> Divide/1
  Saturation1/1 -> Product/2
  Demux/1 -> Interpolation: efficiency2/2, Interpolation: efficiency1/2

== system BugE_v0_40_MAS_loads_reg/Inputs Hardware to Controller/User Inputs/Command Cycles (no regenerative braking assumed) ==
  repeat : Inport
  Time : Inport  Port=2
  drive_cycle : Subsystem
  key : Subsystem
  pedal cycle : Subsystem
  source : Switch  Criteria=u2 > Threshold
  time : Fcn  Expr=rem(u,period)
  use_drive_cycle : Constant  Value=use_drive_cycle  SampleTime=sample_time
  key_out : Outport
  acc_brk_out : Outport  Port=2
  wires:
  time/1 -> drive_cycle/1(time), pedal cycle/2(time), key/1(time)
  Time/1 -> time/1
  repeat/1 -> key/2(repeat), drive_cycle/2(repeat), pedal cycle/3(repeat)
  source/1 -> acc_brk_out/1
  key/2(motor_on) -> pedal cycle/1(motor_on)
  use_drive_cycle/1 -> source/2
  pedal cycle/1(acc/brk) -> source/3
  drive_cycle/1(acc/brk) -> source/1
  [velocity_kph] -> drive_cycle/3(velocity kph)
  key/1(key) -> key_out/1

== system BugE_v0_40_MAS_loads_reg/Inputs Hardware to Controller/User Inputs/key -> ECU bits decode ==
  key : Inport
  Logical Operator : Logic  Operator=OR  AllPortsSameDT=off  OutDataTypeStr=boolean
  accessories (1) : simulink/Logic and Bit Operations/Compare To Constant  relop===  const=1  OutDataTypeStr=boolean
  driving (2) : simulink/Logic and Bit Operations/Compare To Constant  relop===  const=2  OutDataTypeStr=boolean
  ACC : Outport
  IGON : Outport  Port=2
  wires:
  key/1 -> accessories (1)/1, driving (2)/1
  driving (2)/1 -> Logical Operator/1, IGON/1
  accessories (1)/1 -> Logical Operator/2
  Logical Operator/1 -> ACC/1

== system BugE_v0_40_MAS_loads_reg/Inputs Simulation Only/Autopilot load/clock w// pause ==
  In1 : Inport
  Constant1 : Constant  SampleTime=sample_time
  Constant2 : Constant  Value=0  SampleTime=sample_time
  Discrete-Time Integrator : DiscreteIntegrator  gainval=1  InitialConditionSetting=State (most efficient)  SampleTime=sample_time  ICPrevOutput=DiscIntNeverNeededParam  ICPrevScaledInput=DiscIntNeverNeededParam
  Switch1 : Switch  Criteria=u2 > Threshold
  Out1 : Outport
  wires:
  Constant2/1 -> Switch1/3
  In1/1 -> Switch1/2
  Discrete-Time Integrator/1 -> Out1/1
  Switch1/1 -> Discrete-Time Integrator/1
  Constant1/1 -> Switch1/1

== system BugE_v0_40_MAS_loads_reg/Inputs Simulation Only/Command Cycles/drive_cycle ==
  time : Inport
  repeat : Inport  Port=2
  velocity kph : Inport  Port=3
  Add : Sum  Inputs=+-
  Delay : Delay  DelayLength=cyc_avg_time_samples  SampleTime=sample_time
  Discrete PID : simulink/Continuous/PID Controller  Controller=PI  TimeDomain=Discrete-time  SampleTime=sample_time  IntegratorMethod=Forward Euler  FilterMethod=Forward Euler  Form=Parallel  UseFilter=on  ControllerParametersSource=internal  P=0.4  I=0.04  D=0  N=100  InitialConditionSource=internal  InitialConditionForIntegrator=0  InitialConditionForFilter=0  ExternalReset=none  LimitOutput=on  UpperSaturationLimit=1  LowerSaturationLimit=-1  LinearizeAsGain=off  AntiWindupMode=back-calculation  Kb=1  TrackingMode=off  Kt=1  PParamMin=[]  PParamMax=[]  IParamMin=[]  IParamMax=[]  DParamMin=[]  DParamMax=[]  NParamMin=[]  NParamMax=[]  KbParamMin=[]  KbParamMax=[]  KtParamMin=[]  KtParamMax=[]  POutMin=[]  POutMax=[]  IOutMin=[]  IOutMax=[]  DOutMin=[]  DOutMax=[]  NOutMin=[]  NOutMax=[]  KbOutMin=[]  KbOutMax=[]  KtOutMin=[]  KtOutMax=[]  IntegratorOutMin=[]  IntegratorOutMax=[]  FilterOutMin=[]  FilterOutMax=[]  SumOutMin=[]  SumOutMax=[]  SumI1OutMin=[]  SumI1OutMax=[]  SumI2OutMin=[]  SumI2OutMax=[]  SumI3OutMin=[]  SumI3OutMax=[]  SumDOutMin=[]  SumDOutMax=[]  SaturationOutMin=[]  SaturationOutMax=[]  IntegratorContinuousStateAttributes=''  IntegratorStateMustResolveToSignalObject=off  IntegratorRTWStateStorageClass=Auto  FilterContinuousStateAttributes=''  FilterStateMustResolveToSignalObject=off  FilterRTWStateStorageClass=Auto  DifferentiatorICPrevScaledInput=0  DifferentiatorOutMin=[]  DifferentiatorOutMax=[]
  Discrete-Time Integrator1 : DiscreteIntegrator  InitialConditionSetting=State (most efficient)  SampleTime=sample_time  ICPrevOutput=DiscIntNeverNeededParam  ICPrevScaledInput=DiscIntNeverNeededParam
  Dist diff : Scope
  "Dist diff in 10s " : commfilt2/Windowed Integrator  integperiod=sample_time*100*10  roundingMode=Floor  overflowMode=off  InputProcessing=Columns as channels (frame based)
  From Workspace4 : FromWorkspace  VariableName=cyc_kph_ts  SampleTime=sample_time
  Gain : Gain  Gain=-1
  Look-Up Table4 : Lookup_n-D  NumberOfTableDimensions=1  BreakpointsForDimension1=cyc_kph(:,1)  Table=cyc_kph(:,2)  InternalRulePriority=Speed  SaturateOnIntegerOverflow=on  InputSameDT=on
  Mux1 : Mux  Inputs=2
  Mux2 : Mux  Inputs=2
  Unit Delay : UnitDelay  SampleTime=-1
  V diff : Sum  Inputs=+-
  Velocity Tracing : Scope
  acc : Saturate  UpperLimit=1  LowerLimit=0
  brk : Saturate  UpperLimit=0  LowerLimit=-1
  cyc_avg_time_samples : Constant  Value=cyc_avg_time_samples*sample_time  SampleTime=sample_time
  km->m : Gain  Gain=1/360
  vel km/h : Switch  Criteria=u2 > Threshold
  velocity command : Product  Inputs=/*
  acc/brk : Outport
  wires:
  From Workspace4/1 -> vel km/h/3
  Look-Up Table4/1 -> vel km/h/1
  cyc_avg_time_samples/1 -> velocity command/1
  velocity command/1 -> Mux1/1, V diff/1
  vel km/h/1 -> Discrete-Time Integrator1/1
  repeat/1 -> vel km/h/2
  time/1 -> Look-Up Table4/1
  V diff/1 -> "Dist diff in 10s "/1, Discrete PID/1
  Discrete PID/1 -> acc/1, brk/1
  acc/1 -> Mux2/1
  brk/1 -> Gain/1
  velocity kph/1 -> Unit Delay/1
  Gain/1 -> Mux2/2
  Unit Delay/1 -> Mux1/2, V diff/2
  Discrete-Time Integrator1/1 -> Delay/1, Add/1
  Delay/1 -> Add/2
  Add/1 -> velocity command/2
  Mux1/1 -> Velocity Tracing/1
  Mux2/1 -> acc/brk/1
  "Dist diff in 10s "/1 -> km->m/1
  km->m/1 -> Dist diff/1

== system BugE_v0_40_MAS_loads_reg/Inputs Simulation Only/Command Cycles/key ==
  time : Inport
  repeat : Inport  Port=2
  Constant2 : Constant  Value=2  SampleTime=sample_time
  From Workspace3 : FromWorkspace  VariableName=cyc_key_ts  SampleTime=sample_time  Interpolate=off  OutputAfterFinalValue=Holding final value
  Look-Up Table3 : Lookup_n-D  NumberOfTableDimensions=1  BreakpointsForDimension1=cyc_key(:,1)  Table=cyc_key(:,2)  InterpMethod=Flat  InternalRulePriority=Speed  SaturateOnIntegerOverflow=on  InputSameDT=on
  "key " : Switch  Criteria=u2 > Threshold
  motor on : RelationalOperator  Operator===  OutDataTypeStr=boolean
  key : Outport
  motor_on : Outport  Port=2
  wires:
  Look-Up Table3/1 -> "key "/1
  From Workspace3/1 -> "key "/3
  "key "/1 -> key/1, motor on/1
  Constant2/1 -> motor on/2
  motor on/1 -> motor_on/1
  time/1 -> Look-Up Table3/1
  repeat/1 -> "key "/2

== system BugE_v0_40_MAS_loads_reg/Inputs Simulation Only/Command Cycles/pedal cycle ==
  motor_on : Inport
  time : Inport  Port=2
  repeat : Inport  Port=3
  "  1/100" : Gain  Gain=1/100
  1/100 : Gain  Gain=1/100
  Add : Sum  Inputs=+-
  Add1 : Sum  Inputs=+-
  Constant4 : Constant  Value=0  SampleTime=sample_time
  Delay : Delay  DelayLength=cyc_avg_time_samples  SampleTime=sample_time
  Delay1 : Delay  DelayLength=cyc_avg_time_samples  SampleTime=sample_time
  Discrete-Time Integrator : DiscreteIntegrator  InitialConditionSetting=State (most efficient)  SampleTime=sample_time  ICPrevOutput=DiscIntNeverNeededParam  ICPrevScaledInput=DiscIntNeverNeededParam
  Discrete-Time Integrator1 : DiscreteIntegrator  InitialConditionSetting=State (most efficient)  SampleTime=sample_time  ICPrevOutput=DiscIntNeverNeededParam  ICPrevScaledInput=DiscIntNeverNeededParam
  From Workspace : FromWorkspace  VariableName=cyc_acc_ts  SampleTime=sample_time
  From Workspace2 : FromWorkspace  VariableName=cyc_brk_ts  SampleTime=sample_time
  Look-Up Table : Lookup_n-D  NumberOfTableDimensions=1  BreakpointsForDimension1=cyc_acc(:,1)  Table=cyc_acc(:,2)  InternalRulePriority=Speed  SaturateOnIntegerOverflow=on  InputSameDT=on
  Look-Up Table2 : Lookup_n-D  NumberOfTableDimensions=1  BreakpointsForDimension1=cyc_brk(:,1)  Table=cyc_brk(:,2)  InternalRulePriority=Speed  SaturateOnIntegerOverflow=on  InputSameDT=on
  Mux2 : Mux  Inputs=2
  Switch : Switch  Criteria=u2 > Threshold
  Switch3 : Switch  Criteria=u2 > Threshold
  acceleration : Switch  Criteria=u2 > Threshold
  brake : Switch  Criteria=u2 > Threshold
  cyc_avg_time_samples : Constant  Value=cyc_avg_time_samples*sample_time  SampleTime=sample_time
  moving avg acc % : Product  Inputs=/*
  moving avg brk % : Product  Inputs=*/
  acc/brk : Outport
  wires:
  Discrete-Time Integrator1/1 -> Delay1/1, Add/1
  Delay1/1 -> Add/2
  Add/1 -> moving avg acc %/2
  cyc_avg_time_samples/1 -> moving avg acc %/1, moving avg brk %/2
  Look-Up Table/1 -> Switch/1
  From Workspace/1 -> Switch/3
  Discrete-Time Integrator/1 -> Delay/1, Add1/1
  Delay/1 -> Add1/2
  Add1/1 -> moving avg brk %/1
  Look-Up Table2/1 -> Switch3/1
  From Workspace2/1 -> Switch3/3
  "  1/100"/1 -> Discrete-Time Integrator/1
  Switch3/1 -> "  1/100"/1
  1/100/1 -> Discrete-Time Integrator1/1
  Switch/1 -> 1/100/1
  moving avg brk %/1 -> brake/1
  moving avg acc %/1 -> acceleration/1
  Constant4/1 -> acceleration/3, brake/3
  motor_on/1 -> acceleration/2, brake/2
  time/1 -> Look-Up Table/1, Look-Up Table2/1
  repeat/1 -> Switch/2, Switch3/2
  acceleration/1 -> Mux2/1
  Mux2/1 -> acc/brk/1
  brake/1 -> Mux2/2

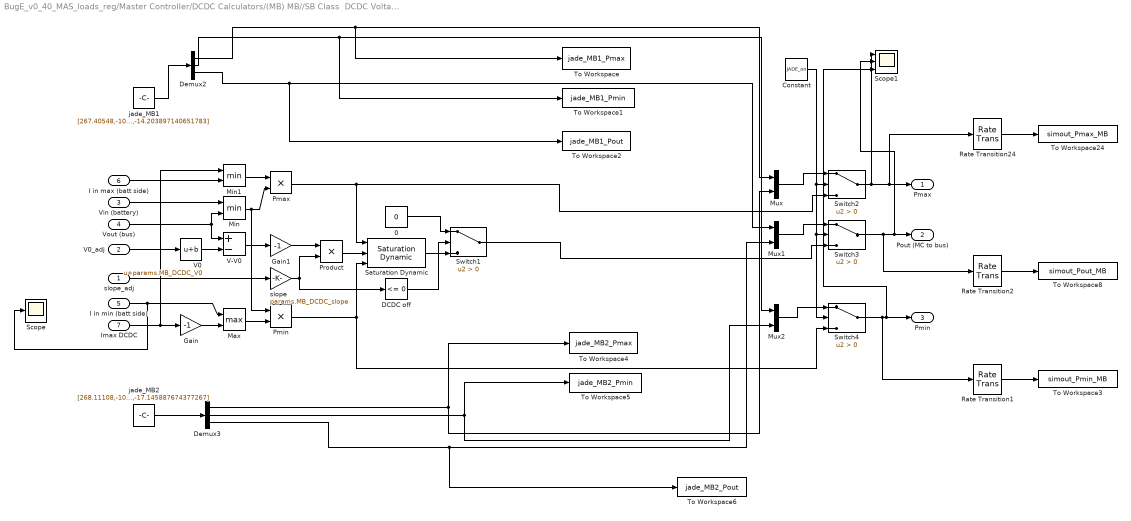
== system BugE_v0_40_MAS_loads_reg/Master Controller/DCDC Calculators/(MB) MB//SB Class  DCDC Voltage => Power Droop ==
  slope_adj : Inport
  V0_adj : Inport  Port=2
  Vin (battery) : Inport  Port=3
  Vout (bus) : Inport  Port=4
  I in min (batt side) : Inport  Port=5
  I in max (batt side) : Inport  Port=6
  Imax DCDC : Inport  Port=7
  0 : Constant  Value=0  SampleTime=sample_time
  Constant : Constant  Value=JADE_on
  DCDC off : simulink/Logic and Bit Operations/Compare To Zero  relop=<=  OutDataTypeStr=boolean
  Demux2 : Demux  Outputs=3
  Demux3 : Demux  Outputs=3
  Gain : Gain  Gain=-1
  Gain1 : Gain  Gain=-1
  Max : MinMax  Function=max  Inputs=2
  Min : MinMax  Inputs=2
  Min1 : MinMax  Inputs=2
  Mux : Mux  Inputs=2
  Mux1 : Mux  Inputs=2
  Mux2 : Mux  Inputs=2
  Pmax : Product  Inputs=**
  Pmin : Product  Inputs=**
  Product : Product
  Rate Transition1 : RateTransition
  Rate Transition2 : RateTransition
  Rate Transition24 : RateTransition
  Saturation Dynamic : simulink/Discontinuities/Saturation Dynamic  OutMin=[]  OutMax=[]  OutDataTypeStr=Inherit: Same as second input  OutDataType=fixdt(1, 16)  OutScaling=2^-10  DoSatur=off
  Scope : Scope
  Scope1 : Scope  NumInputPorts=3
  Switch{1..4} (4 alike) : Switch  Criteria=u2 > Threshold
  To Workspace : ToWorkspace  VariableName=jade_MB1_Pmax  SaveFormat=Timeseries  SampleTime=-1
  To Workspace1 : ToWorkspace  VariableName=jade_MB1_Pmin  SaveFormat=Timeseries  SampleTime=-1
  To Workspace2 : ToWorkspace  VariableName=jade_MB1_Pout  SaveFormat=Timeseries  SampleTime=-1
  To Workspace24 : ToWorkspace  VariableName=simout_Pmax_MB  SampleTime=1
      settings: MaxDataPoints=Inf
  To Workspace3 : ToWorkspace  VariableName=simout_Pmin_MB  SampleTime=1
      settings: MaxDataPoints=Inf
  To Workspace4 : ToWorkspace  VariableName=jade_MB2_Pmax  SaveFormat=Timeseries  SampleTime=-1
  To Workspace5 : ToWorkspace  VariableName=jade_MB2_Pmin  SaveFormat=Timeseries  SampleTime=-1
  To Workspace6 : ToWorkspace  VariableName=jade_MB2_Pout  SaveFormat=Timeseries  SampleTime=-1
  To Workspace8 : ToWorkspace  VariableName=simout_Pout_MB  SampleTime=1
      settings: MaxDataPoints=Inf
  V-V0 : Sum  Inputs=+-
  V0 : Bias  Bias=params.MB_DCDC_V0
  jade_MB1 : Constant  Value=[267.40548,-103.31723246970002,-14.203897140651783]  SampleTime=sample_time
  jade_MB2 : Constant  Value=[268.11108,-103.56684168600002,-17.145887674377267]  SampleTime=sample_time
  slope : Gain  Gain=params.MB_DCDC_slope
  " Pmax " : Outport
  Pout (MC to bus) : Outport  Port=2
  " Pmin " : Outport  Port=3
  wires:
  Vout (bus)/1 -> V-V0/1, Min/2
  Pmin/1 -> Saturation Dynamic/3, Switch4/3
  Switch1/1 -> Switch3/3
  Saturation Dynamic/1 -> Switch1/3
  0/1 -> Switch1/1
  V0_adj/1 -> V0/1
  Vin (battery)/1 -> Min/1
  Min/1 -> Pmax/2, Pmin/1
  Pmax/1 -> Switch2/3, Saturation Dynamic/1
  I in max (batt side)/1 -> Min1/2
  Min1/1 -> Pmax/1
  Imax DCDC/1 -> Gain/1, Min1/1
  Gain/1 -> Max/2
  I in min (batt side)/1 -> Scope/1, Max/1
  Max/1 -> Pmin/2
  V-V0/1 -> Gain1/1
  slope_adj/1 -> slope/1
  Gain1/1 -> Product/1
  slope/1 -> Product/2, DCDC off/1
  Product/1 -> Saturation Dynamic/2
  V0/1 -> V-V0/2
  jade_MB1/1 -> Demux2/1
  Demux2/1 -> To Workspace/1, Mux/1
  Demux2/2 -> To Workspace1/1, Mux2/1
  Demux2/3 -> To Workspace2/1, Mux1/1
  jade_MB2/1 -> Demux3/1
  Demux3/1 -> Mux/2, To Workspace4/1
  Demux3/2 -> Mux2/2, To Workspace5/1
  Demux3/3 -> To Workspace6/1, Mux1/2
  Mux/1 -> Switch2/1
  Switch3/1 -> Rate Transition2/1, Scope1/2, Pout (MC to bus)/1
  Constant/1 -> Switch4/2, Switch3/2, Switch2/2
  Switch2/1 -> Scope1/1, Rate Transition24/1, " Pmax "/1
  Mux1/1 -> Switch3/1
  Mux2/1 -> Switch4/1
  Rate Transition24/1 -> To Workspace24/1
  Switch4/1 -> Rate Transition1/1, Scope1/3, " Pmin "/1
  Rate Transition1/1 -> To Workspace3/1
  Rate Transition2/1 -> To Workspace8/1
  DCDC off/1 -> Switch1/2

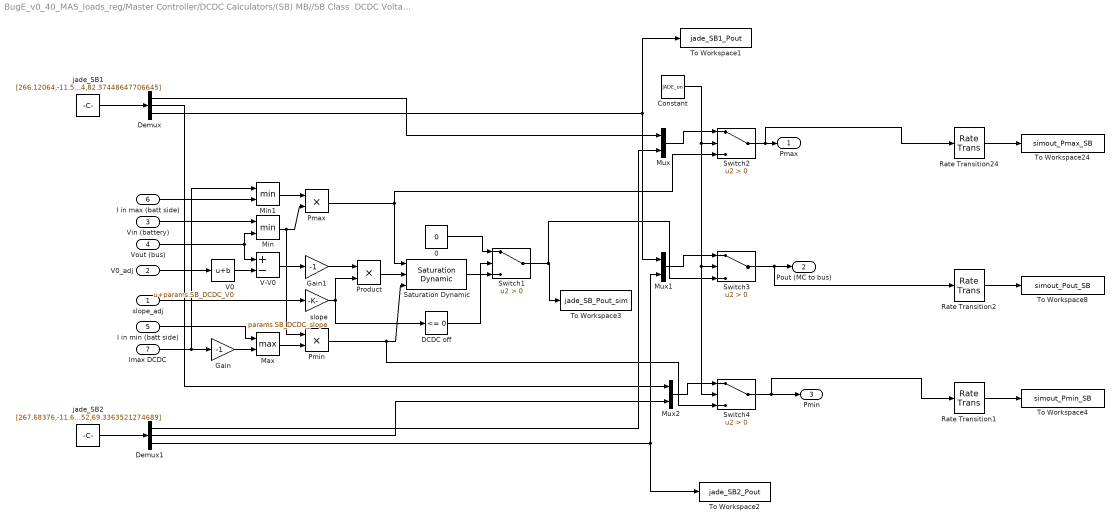
== system BugE_v0_40_MAS_loads_reg/Master Controller/DCDC Calculators/(SB) MB//SB Class  DCDC Voltage => Power Droop1 ==
  slope_adj : Inport
  V0_adj : Inport  Port=2
  Vin (battery) : Inport  Port=3
  Vout (bus) : Inport  Port=4
  I in min (batt side) : Inport  Port=5
  I in max (batt side) : Inport  Port=6
  Imax DCDC : Inport  Port=7
  0 : Constant  Value=0  SampleTime=sample_time
  Constant : Constant  Value=JADE_on
  DCDC off : simulink/Logic and Bit Operations/Compare To Zero  relop=<=  OutDataTypeStr=boolean
  Demux : Demux  Outputs=3
  Demux1 : Demux  Outputs=3
  Gain : Gain  Gain=-1
  Gain1 : Gain  Gain=-1
  Max : MinMax  Function=max  Inputs=2
  Min : MinMax  Inputs=2
  Min1 : MinMax  Inputs=2
  Mux : Mux  Inputs=2
  Mux1 : Mux  Inputs=2
  Mux2 : Mux  Inputs=2
  Pmax : Product  Inputs=**
  Pmin : Product  Inputs=**
  Product : Product
  Rate Transition1 : RateTransition
  Rate Transition2 : RateTransition
  Rate Transition24 : RateTransition
  Saturation Dynamic : simulink/Discontinuities/Saturation Dynamic  OutMin=[]  OutMax=[]  OutDataTypeStr=Inherit: Same as second input  OutDataType=fixdt(1, 16)  OutScaling=2^-10  DoSatur=off
  Switch{1..4} (4 alike) : Switch  Criteria=u2 > Threshold
  To Workspace1 : ToWorkspace  VariableName=jade_SB1_Pout  SaveFormat=Timeseries  SampleTime=-1
  To Workspace2 : ToWorkspace  VariableName=jade_SB2_Pout  SaveFormat=Timeseries  SampleTime=-1
  To Workspace24 : ToWorkspace  VariableName=simout_Pmax_SB  SampleTime=1
      settings: MaxDataPoints=Inf
  To Workspace3 : ToWorkspace  VariableName=jade_SB_Pout_sim  SaveFormat=Timeseries  SampleTime=-1
  To Workspace4 : ToWorkspace  VariableName=simout_Pmin_SB  SampleTime=1
      settings: MaxDataPoints=Inf
  To Workspace8 : ToWorkspace  VariableName=simout_Pout_SB  SampleTime=1
      settings: MaxDataPoints=Inf
  V-V0 : Sum  Inputs=+-
  V0 : Bias  Bias=params.SB_DCDC_V0
  jade_SB1 : Constant  Value=[266.12064,-11.5633853424,82.37448647706645]  SampleTime=sample_time
  jade_SB2 : Constant  Value=[267.68376,-11.6384437452,69.3363521274689]  SampleTime=sample_time
  slope : Gain  Gain=params.SB_DCDC_slope
  " Pmax " : Outport
  Pout (MC to bus) : Outport  Port=2
  " Pmin" : Outport  Port=3
  wires:
  Vout (bus)/1 -> V-V0/1, Min/2
  Pmin/1 -> Switch4/3, Saturation Dynamic/3
  Switch1/1 -> Switch3/3, To Workspace3/1
  Saturation Dynamic/1 -> Switch1/3
  0/1 -> Switch1/1
  V0_adj/1 -> V0/1
  Vin (battery)/1 -> Min/1
  Min/1 -> Pmax/2, Pmin/1
  I in max (batt side)/1 -> Min1/2
  Min1/1 -> Pmax/1
  Imax DCDC/1 -> Gain/1, Min1/1
  Gain/1 -> Max/2
  I in min (batt side)/1 -> Max/1
  Max/1 -> Pmin/2
  V-V0/1 -> Gain1/1
  slope_adj/1 -> slope/1
  Gain1/1 -> Product/1
  slope/1 -> Product/2, DCDC off/1
  Product/1 -> Saturation Dynamic/2
  DCDC off/1 -> Switch1/2
  V0/1 -> V-V0/2
  jade_SB1/1 -> Demux/1
  jade_SB2/1 -> Demux1/1
  Demux/1 -> Mux/1
  Demux/2 -> Mux2/1
  Demux/3 -> Mux1/1, To Workspace1/1
  Demux1/1 -> Mux/2
  Demux1/2 -> Mux2/2
  Demux1/3 -> Mux1/2, To Workspace2/1
  Pmax/1 -> Switch2/3, Saturation Dynamic/1
  Constant/1 -> Switch2/2, Switch3/2, Switch4/2
  Mux/1 -> Switch2/1
  Mux1/1 -> Switch3/1
  Mux2/1 -> Switch4/1
  Switch3/1 -> Rate Transition2/1, Pout (MC to bus)/1
  Switch2/1 -> Rate Transition24/1, " Pmax "/1
  Rate Transition24/1 -> To Workspace24/1
  Switch4/1 -> Rate Transition1/1, " Pmin"/1
  Rate Transition1/1 -> To Workspace4/1
  Rate Transition2/1 -> To Workspace8/1

== system BugE_v0_40_MAS_loads_reg/Master Controller/DCDC Calculators/FE // CHG Class Voltage => Power Droop ==
  Vbus_min : Inport
  Vbus_max : Inport  Port=2
  Vbus : Inport  Port=3
  Pmax_spec : Inport  Port=4
  50ms moving avg : DiscreteFir  Coefficients=ones(1,0.05*(1/sample_time))/(0.05*(1/sample_time))  SampleTime=sample_time
  >=0 : Saturate  UpperLimit=inf  LowerLimit=0
  Constant6 : Constant  SampleTime=sample_time
  Divide : Product  Inputs=*/
  Product : Product
  Subtract1 : Sum  Inputs=+-
  Subtract2 : Sum  Inputs=++-
  Subtract3 : Sum  Inputs=+-
  Subtract4 : Sum  Inputs=+-
  Subtract5 : Sum  Inputs=-+
  "[0,1]" : Saturate  UpperLimit=1-eps  LowerLimit=0
  beta : Constant  Value=0.9  SampleTime=sample_time
  sqr : Math  Operator=square  SaturateOnIntegerOverflow=on
  vf : Product  Inputs=*/
  Pmax_lim : Outport
  wires:
  Product/1 -> >=0/1
  Divide/1 -> Subtract2/3
  beta/1 -> Subtract3/2
  Subtract3/1 -> sqr/1
  sqr/1 -> Subtract2/2, Divide/1
  Constant6/1 -> Subtract2/1, Subtract3/1, Subtract4/1
  vf/1 -> "[0,1]"/1
  Subtract4/1 -> Divide/2
  >=0/1 -> Pmax_lim/1
  Vbus/1 -> 50ms moving avg/1
  Vbus_min/1 -> Subtract5/1, Subtract1/2
  Vbus_max/1 -> Subtract5/2
  Subtract5/1 -> vf/2
  Subtract1/1 -> vf/1
  "[0,1]"/1 -> Subtract4/2
  Subtract2/1 -> Product/1
  Pmax_spec/1 -> Product/2
  50ms moving avg/1 -> Subtract1/1

== system BugE_v0_40_MAS_loads_reg/Master Controller/DCDC Calculators/LD Class Voltage => Power Droop ==
  Vbus_min : Inport
  Vbus_max : Inport  Port=2
  Vbus : Inport  Port=3
  Pmax_spec_abs : Inport  Port=4
  50ms moving avg : DiscreteFir  Commented=through  Coefficients=ones(1,0.05*(1/sample_time))/(0.05*(1/sample_time))  SampleTime=sample_time
  <=0 : Saturate  UpperLimit=0  LowerLimit=-inf
  Constant6 : Constant  SampleTime=sample_time
  Divide1 : Product  Inputs=*/
  Product : Product
  Scope : Scope  NumInputPorts=2
  Subtract : Sum  Inputs=--+
  Subtract1 : Sum  Inputs=+-
  Subtract2 : Sum  Inputs=+-
  Subtract5 : Sum  Inputs=-+
  "[0,1]" : Saturate  UpperLimit=1  LowerLimit=eps
  beta : Constant  Value=0.9  SampleTime=sample_time
  sqr : Math  Operator=square  SaturateOnIntegerOverflow=on
  vf : Product  Inputs=*/
  Pmax_lim (neg) : Outport
  wires:
  vf/1 -> Scope/1, "[0,1]"/1
  50ms moving avg/1 -> Subtract1/1
  Vbus_min/1 -> Subtract5/1, Subtract1/2
  Vbus_max/1 -> Subtract5/2
  Subtract5/1 -> vf/2
  Subtract1/1 -> vf/1
  Constant6/1 -> Subtract/1, Subtract2/1
  beta/1 -> Subtract2/2
  Divide1/1 -> Subtract/3
  Subtract2/1 -> sqr/1
  sqr/1 -> Subtract/2, Divide1/1
  "[0,1]"/1 -> Divide1/2
  <=0/1 -> Scope/2, Pmax_lim (neg)/1
  Subtract/1 -> Product/1
  Pmax_spec_abs/1 -> Product/2
  Product/1 -> <=0/1
  Vbus/1 -> 50ms moving avg/1

== system BugE_v0_40_MAS_loads_reg/Master Controller/DCDC Calculators/ones voltage cmd ==
  I : Inport
  2dbl : DataTypeConversion
  Bias : Bias  Bias=1
  Gain : Gain  Gain=0
  O : Outport
  wires:
  Gain/1 -> Bias/1
  I/1 -> 2dbl/1
  2dbl/1 -> Gain/1
  Bias/1 -> O/1

== system BugE_v0_40_MAS_loads_reg/Master Controller/DCDC Calculators/zeros power cmd ==
  I : Inport
  2dbl : DataTypeConversion
  Gain : Gain  Gain=0
  O : Outport
  wires:
  Gain/1 -> O/1
  I/1 -> 2dbl/1
  2dbl/1 -> Gain/1

== system BugE_v0_40_MAS_loads_reg/Master Controller/DCDC Calculators/zeros power cmd1 ==
  I : Inport
  2dbl : DataTypeConversion
  Gain : Gain  Gain=0
  O : Outport
  wires:
  Gain/1 -> O/1
  I/1 -> 2dbl/1
  2dbl/1 -> Gain/1

== system BugE_v0_40_MAS_loads_reg/Master Controller/Motor Controller/MB Class Current => Throttle Droop ==
  I : Inport
  Imax : Inport  Port=2
  Constant6 : Constant  SampleTime=sample_time
  Divide : Product  Inputs=*/
  If : Product  Inputs=*/
  Rate Limiter 0-full in 1s : RateLimiter  FallingSlewLimit=-1/sample_time  SampleTimeMode=inherited  LinearizeAsGain=off
  Subtract2 : Sum  Inputs=++-
  Subtract3 : Sum  Inputs=+-
  Subtract4 : Sum  Inputs=+-
  "[0, 1]" : Saturate  UpperLimit=1-eps  LowerLimit=0
  "[0,1-eps]" : Saturate  UpperLimit=1-eps  LowerLimit=0
  beta : Constant  Value=0.85  SampleTime=sample_time
  moving average 200ms : DiscreteFir  Coefficients=ones(1,20)/20  SampleTime=sample_time
  sqr : Math  Operator=square  SaturateOnIntegerOverflow=on
  thr_max_lim : Outport
  wires:
  Subtract2/1 -> "[0, 1]"/1
  Divide/1 -> Subtract2/3
  beta/1 -> Subtract3/2
  Subtract3/1 -> sqr/1
  sqr/1 -> Subtract2/2, Divide/1
  Constant6/1 -> Subtract2/1, Subtract3/1, Subtract4/1
  Subtract4/1 -> Divide/2
  "[0,1-eps]"/1 -> Subtract4/2
  Imax/1 -> If/2
  If/1 -> "[0,1-eps]"/1
  "[0, 1]"/1 -> Rate Limiter 0-full in 1s/1
  Rate Limiter 0-full in 1s/1 -> moving average 200ms/1
  moving average 200ms/1 -> thr_max_lim/1
  I/1 -> If/1
